simulink model "power_OLTCregtransformer"  (Simulink 6.0)
settings: Solver=ode23tb  StartTime=0.0  StopTime=120  MaxStep=1/60  RelTol=1e-4  AbsTol=1e-3
libraries: powerlib x75, powerlib_extras x18, simulink_extras x1
(part 2 of 3)

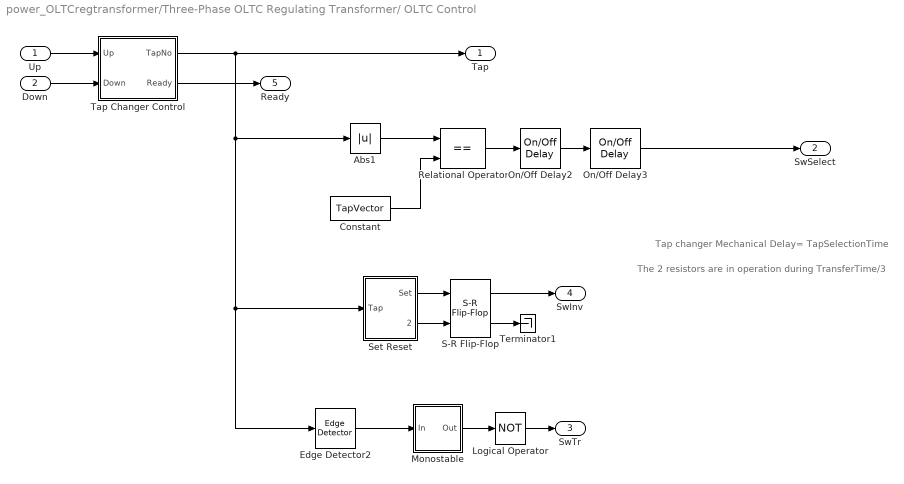
== system power_OLTCregtransformer/Three-Phase OLTC Regulating Transformer/ OLTC Control ==
  note: The 2 resistors are in operation during TransferTime/3
  note: Tap changer Mechanical Delay= TapSelectionTime
  Up : Inport  Port=1  LatchInput=off
  Down : Inport  Port=2  LatchInput=off
  Abs1 : Abs  SaturateOnIntegerOverflow=on
  Constant : Constant  Value=TapVector
  Edge Detector2 : powerlib_extras/Control  Blocks/Edge Detector  model=Either  ic=0
  Logical Operator : Logic  Operator=NOT  AllPortsSameDT=off
  Monostable : Subsystem  mask(Monostable Flip-Flop){EdgeDetect=Rising, t_mono=TransferTime, ic=1}
      mask prompts: EdgeDetect "Edge detection"; t_mono "Pulse duration (s):"; ic "Input at t = -eps:"
      mask help:
      | After being triggered  by the specified edge (Rising, Falling or Either), this block outputs a pulse (TRUE signal) for the time specified by parameter "Pulse duration".
      | If the specified edge is detected while the output is TRUE, the monostable is not retriggered
      |
      | The input value (0/1) at time preceeding t = 0 is specified by the parameter "input at t = -eps.
      mask init:
      | str=sprintf('%g %c',t_mono,'s');
      | if (EdgeDetect ~=3)
      |     x1 = (EdgeDetect -1)*10;
      |     x2 = (EdgeDetect -1)*30;
      | 	X1=[15-8,25,25,35+8]+0; Y1=[65+x2,65+x2,95-x2,95-x2];
      | 	X2=[15,25,35]+0;   Y2=[75+x1,85-x1,75+x1];
      | 	X3=[];X4=[];Y3=[];Y4=[];	
      | else
      | 	x1 = 10;
      | 	x2 = 30;
      | 	X1=[15,25,25,35]-14;  Y1=[65,65,95,95];
      | 	X2=[15,25,35]-14;    Y2=[75,85,75];
      | 	X3=[15,25,25,35]+14; Y3=[65+x2,65+x2,95-x2,95-x2];
      | 	X4=[15,25,35]+14;   Y4=[75+x1,85-x1,75+x1];
      | end
      mask StyleString: popup(Rising|Falling|Either),edit,edit
      mask Display:
      | plot(0,0,100,100,[100 75 75 25 25 0],[25 25 50 50 25 25]-0,X1,Y1,X2,Y2,X3,Y3,X4,Y4);
      | text(45,37,'T');
      | text(15,15,str);
  On/Off Delay2 : powerlib_extras/Control  Blocks/On//Off Delay  type_delay=On delay  delay=TransferTime/3  ic=1
  On/Off Delay3 : powerlib_extras/Control  Blocks/On//Off Delay  type_delay=Off delay  delay=2*TransferTime/3  ic=InitialStates
  Relational Operator : RelationalOperator  Operator===
  S-R Flip-Flop : simulink_extras/Flip Flops/S-R Flip-Flop  initial_condition=InitialTap>=0
  Set Reset : Subsystem
  Tap Changer Control : Subsystem  mask(Tap Changer Control){MinMaxTap=[-NumberOfTaps  +NumberOfTaps], InitialPosition=InitialTap, MecDelay=TapSelectionTime}
      mask prompts: MinMaxTap "Minimum and maximum tap number [ Min  Max ] :"; InitialPosition "Initial tap position"; MecDelay "Mechanical delay time"
      mask init:
      | if MecDelay<=0,
      | 	MecDelay=1/60;
      | end
  Terminator1 : Terminator
  Tap : Outport
  SwSelect : Outport  Port=2
  SwTr : Outport  Port=3
  SwInv : Outport  Port=4
  Ready : Outport  Port=5
  wires:
  On/Off Delay3/1 -> SwSelect/1
  Constant/1 -> Relational Operator/2
  Logical Operator/1 -> SwTr/1
  Down/1 -> Tap Changer Control/2(Down)
  Up/1 -> Tap Changer Control/1(Up)
  Relational Operator/1 -> On/Off Delay2/1
  On/Off Delay2/1 -> On/Off Delay3/1
  Monostable/1(Out) -> Logical Operator/1
  Tap Changer Control/1(TapNo) -> Tap/1, Edge Detector2/1, Set Reset/1(Tap), Abs1/1
  Tap Changer Control/2(Ready) -> Ready/1
  S-R Flip-Flop/2 -> Terminator1/1
  Set Reset/1(Set) -> S-R Flip-Flop/1
  Set Reset/2(Reset) -> S-R Flip-Flop/2
  Edge Detector2/1 -> Monostable/1(In)
  S-R Flip-Flop/1 -> SwInv/1
  Abs1/1 -> Relational Operator/1

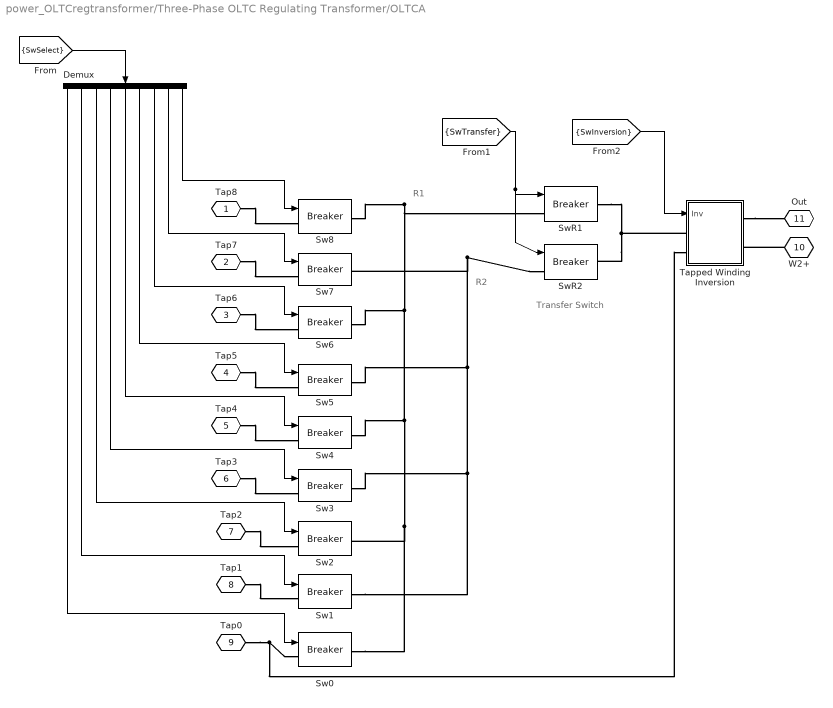
== system power_OLTCregtransformer/Three-Phase OLTC Regulating Transformer/OLTCA ==
  note: R2
  note: R1
  note: Transfer Switch
  Demux : Demux  Orientation=down  Outputs=9
  "Sw0 " : powerlib/Elements/Breaker  BreakerResistance=1e-4  InitialState=InitialStates(1)  SnubberResistance=1e6  SnubberCapacitance=inf  SwitchingTimes="[ 1/60  5/60 ]"  External=on  Measurements=None
  "Sw1 " : powerlib/Elements/Breaker  BreakerResistance=1e-4  InitialState=InitialStates(2)  SnubberResistance=1e6  SnubberCapacitance=inf  SwitchingTimes="[ 1/60  5/60 ]"  External=on  Measurements=None
  "Sw2 " : powerlib/Elements/Breaker  BreakerResistance=1e-4  InitialState=InitialStates(3)  SnubberResistance=1e6  SnubberCapacitance=inf  SwitchingTimes="[ 1/60  5/60 ]"  External=on  Measurements=None
  "Sw3 " : powerlib/Elements/Breaker  BreakerResistance=1e-4  InitialState=InitialStates(4)  SnubberResistance=1e6  SnubberCapacitance=inf  SwitchingTimes="[ 1/60  5/60 ]"  External=on  Measurements=None
  "Sw4 " : powerlib/Elements/Breaker  BreakerResistance=1e-4  InitialState=InitialStates(5)  SnubberResistance=1e6  SnubberCapacitance=inf  SwitchingTimes="[ 1/60  5/60 ]"  External=on  Measurements=None
  "Sw5 " : powerlib/Elements/Breaker  BreakerResistance=1e-4  InitialState=InitialStates(6)  SnubberResistance=1e6  SnubberCapacitance=inf  SwitchingTimes="[ 1/60  5/60 ]"  External=on  Measurements=None
  "Sw6 " : powerlib/Elements/Breaker  BreakerResistance=1e-4  InitialState=InitialStates(7)  SnubberResistance=1e6  SnubberCapacitance=inf  SwitchingTimes="[ 1/60  5/60 ]"  External=on  Measurements=None
  "Sw7 " : powerlib/Elements/Breaker  BreakerResistance=1e-4  InitialState=InitialStates(8)  SnubberResistance=1e6  SnubberCapacitance=inf  SwitchingTimes="[ 1/60  5/60 ]"  External=on  Measurements=None
  "Sw8 " : powerlib/Elements/Breaker  BreakerResistance=1e-4  InitialState=InitialStates(9)  SnubberResistance=1e6  SnubberCapacitance=inf  SwitchingTimes="[ 1/60  5/60 ]"  External=on  Measurements=None
  SwR1 : powerlib/Elements/Breaker  BreakerResistance=1e-4  InitialState=1  SnubberResistance=Rtransfer  SnubberCapacitance=inf  SwitchingTimes="[ 1/60  5/60 ]"  External=on  Measurements=None
  SwR2 : powerlib/Elements/Breaker  BreakerResistance=1e-4  InitialState=1  SnubberResistance=Rtransfer  SnubberCapacitance=inf  SwitchingTimes="[ 1/60  5/60 ]"  External=on  Measurements=None
  Tapped Winding Inversion : Subsystem
  Tap8 : PMIOPort  Port=1  Side=Right
  Tap7 : PMIOPort  Port=2  Side=Right
  Tap6 : PMIOPort  Port=3  Side=Right
  Tap5 : PMIOPort  Port=4  Side=Right
  Tap4 : PMIOPort  Port=5  Side=Right
  Tap3 : PMIOPort  Port=6  Side=Right
  Tap2 : PMIOPort  Port=7  Side=Right
  Tap1 : PMIOPort  Port=8  Side=Right
  Tap0 : PMIOPort  Port=9  Side=Right
  W2+ : PMIOPort  Orientation=left  Port=10  Side=Right
  Out : PMIOPort  Orientation=left  Port=11  Side=Left
  wires:
  Demux/9 -> "Sw8 "/1
  Demux/8 -> "Sw7 "/1
  Demux/7 -> "Sw6 "/1
  Demux/6 -> "Sw5 "/1
  Demux/5 -> "Sw4 "/1
  Demux/4 -> "Sw3 "/1
  Demux/3 -> "Sw2 "/1
  Demux/2 -> "Sw1 "/1
  Demux/1 -> "Sw0 "/1
  [SwInversion] -> Tapped Winding Inversion/1(Inv)
  [SwTransfer] -> SwR2/1, SwR1/1
  [SwSelect] -> Demux/1
  connections:
  "Sw0 "/LConn1 -- Tap0/RConn1 -- Tapped Winding Inversion/LConn2
  Tap1/RConn1 -- "Sw1 "/LConn1
  Tap2/RConn1 -- "Sw2 "/LConn1
  Tap6/RConn1 -- "Sw6 "/LConn1
  Tap4/RConn1 -- "Sw4 "/LConn1
  Tap5/RConn1 -- "Sw5 "/LConn1
  SwR1/RConn1 -- Tapped Winding Inversion/LConn1 -- SwR2/RConn1
  SwR2/LConn1 -- "Sw7 "/RConn1 -- "Sw5 "/RConn1 -- "Sw3 "/RConn1 -- "Sw1 "/RConn1
  Tapped Winding Inversion/RConn1 -- Out/RConn1
  W2+/RConn1 -- Tapped Winding Inversion/RConn2
  "Sw6 "/RConn1 -- "Sw4 "/RConn1 -- "Sw2 "/RConn1 -- "Sw0 "/RConn1 -- "Sw8 "/RConn1 -- SwR1/LConn1
  Tap3/RConn1 -- "Sw3 "/LConn1
  Tap8/RConn1 -- "Sw8 "/LConn1
  Tap7/RConn1 -- "Sw7 "/LConn1

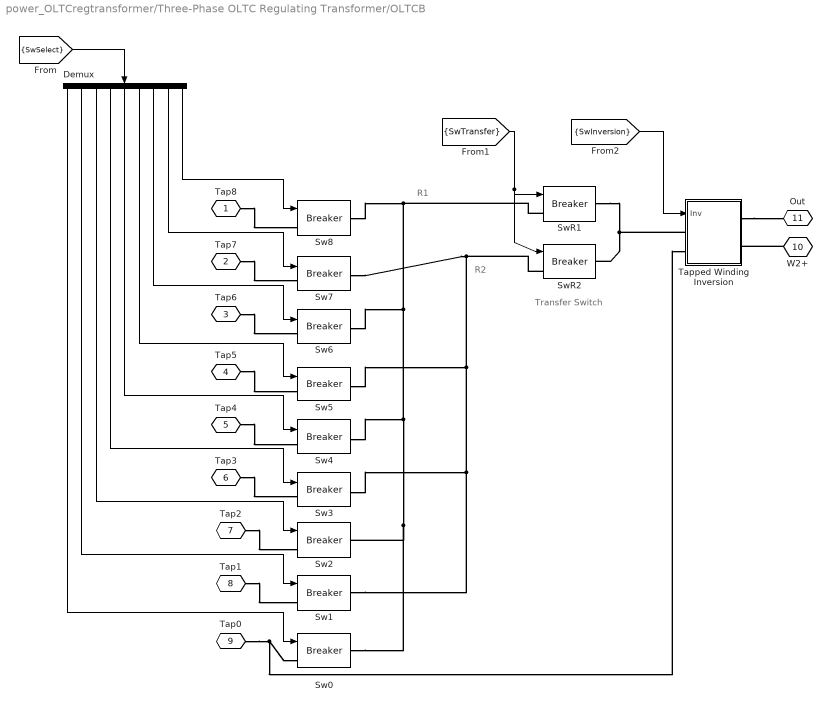
== system power_OLTCregtransformer/Three-Phase OLTC Regulating Transformer/OLTCB ==
  note: Transfer Switch
  note: R1
  note: R2
  Demux : Demux  Orientation=down  Outputs=9
  "Sw0 " : powerlib/Elements/Breaker  BreakerResistance=1e-4  InitialState=InitialStates(1)  SnubberResistance=1e6  SnubberCapacitance=inf  SwitchingTimes="[ 1/60  5/60 ]"  External=on  Measurements=None
  "Sw1 " : powerlib/Elements/Breaker  BreakerResistance=1e-4  InitialState=InitialStates(2)  SnubberResistance=1e6  SnubberCapacitance=inf  SwitchingTimes="[ 1/60  5/60 ]"  External=on  Measurements=None
  "Sw2 " : powerlib/Elements/Breaker  BreakerResistance=1e-4  InitialState=InitialStates(3)  SnubberResistance=1e6  SnubberCapacitance=inf  SwitchingTimes="[ 1/60  5/60 ]"  External=on  Measurements=None
  "Sw3 " : powerlib/Elements/Breaker  BreakerResistance=1e-4  InitialState=InitialStates(4)  SnubberResistance=1e6  SnubberCapacitance=inf  SwitchingTimes="[ 1/60  5/60 ]"  External=on  Measurements=None
  "Sw4 " : powerlib/Elements/Breaker  BreakerResistance=1e-4  InitialState=InitialStates(5)  SnubberResistance=1e6  SnubberCapacitance=inf  SwitchingTimes="[ 1/60  5/60 ]"  External=on  Measurements=None
  "Sw5 " : powerlib/Elements/Breaker  BreakerResistance=1e-4  InitialState=InitialStates(6)  SnubberResistance=1e6  SnubberCapacitance=inf  SwitchingTimes="[ 1/60  5/60 ]"  External=on  Measurements=None
  "Sw6 " : powerlib/Elements/Breaker  BreakerResistance=1e-4  InitialState=InitialStates(7)  SnubberResistance=1e6  SnubberCapacitance=inf  SwitchingTimes="[ 1/60  5/60 ]"  External=on  Measurements=None
  "Sw7 " : powerlib/Elements/Breaker  BreakerResistance=1e-4  InitialState=InitialStates(8)  SnubberResistance=1e6  SnubberCapacitance=inf  SwitchingTimes="[ 1/60  5/60 ]"  External=on  Measurements=None
  "Sw8 " : powerlib/Elements/Breaker  BreakerResistance=1e-4  InitialState=InitialStates(9)  SnubberResistance=1e6  SnubberCapacitance=inf  SwitchingTimes="[ 1/60  5/60 ]"  External=on  Measurements=None
  SwR1 : powerlib/Elements/Breaker  BreakerResistance=1e-4  InitialState=1  SnubberResistance=Rtransfer  SnubberCapacitance=inf  SwitchingTimes="[ 1/60  5/60 ]"  External=on  Measurements=None
  SwR2 : powerlib/Elements/Breaker  BreakerResistance=1e-4  InitialState=1  SnubberResistance=Rtransfer  SnubberCapacitance=inf  SwitchingTimes="[ 1/60  5/60 ]"  External=on  Measurements=None
  Tapped Winding Inversion : Subsystem
  Tap8 : PMIOPort  Port=1  Side=Right
  Tap7 : PMIOPort  Port=2  Side=Right
  Tap6 : PMIOPort  Port=3  Side=Right
  Tap5 : PMIOPort  Port=4  Side=Right
  Tap4 : PMIOPort  Port=5  Side=Right
  Tap3 : PMIOPort  Port=6  Side=Right
  Tap2 : PMIOPort  Port=7  Side=Right
  Tap1 : PMIOPort  Port=8  Side=Right
  Tap0 : PMIOPort  Port=9  Side=Right
  W2+ : PMIOPort  Orientation=left  Port=10  Side=Right
  Out : PMIOPort  Orientation=left  Port=11  Side=Left
  wires:
  [SwSelect] -> Demux/1
  [SwTransfer] -> SwR1/1, SwR2/1
  [SwInversion] -> Tapped Winding Inversion/1(Inv)
  Demux/1 -> "Sw0 "/1
  Demux/2 -> "Sw1 "/1
  Demux/3 -> "Sw2 "/1
  Demux/4 -> "Sw3 "/1
  Demux/5 -> "Sw4 "/1
  Demux/6 -> "Sw5 "/1
  Demux/7 -> "Sw6 "/1
  Demux/8 -> "Sw7 "/1
  Demux/9 -> "Sw8 "/1
  connections:
  Tap7/RConn1 -- "Sw7 "/LConn1
  Tap8/RConn1 -- "Sw8 "/LConn1
  Tap3/RConn1 -- "Sw3 "/LConn1
  "Sw0 "/RConn1 -- "Sw4 "/RConn1 -- SwR1/LConn1 -- "Sw8 "/RConn1 -- "Sw6 "/RConn1 -- "Sw2 "/RConn1
  W2+/RConn1 -- Tapped Winding Inversion/RConn2
  Tapped Winding Inversion/RConn1 -- Out/RConn1
  "Sw1 "/RConn1 -- "Sw3 "/RConn1 -- SwR2/LConn1 -- "Sw7 "/RConn1 -- "Sw5 "/RConn1
  SwR2/RConn1 -- Tapped Winding Inversion/LConn1 -- SwR1/RConn1
  Tap5/RConn1 -- "Sw5 "/LConn1
  Tap4/RConn1 -- "Sw4 "/LConn1
  Tap6/RConn1 -- "Sw6 "/LConn1
  Tap2/RConn1 -- "Sw2 "/LConn1
  Tap1/RConn1 -- "Sw1 "/LConn1
  "Sw0 "/LConn1 -- Tapped Winding Inversion/LConn2 -- Tap0/RConn1

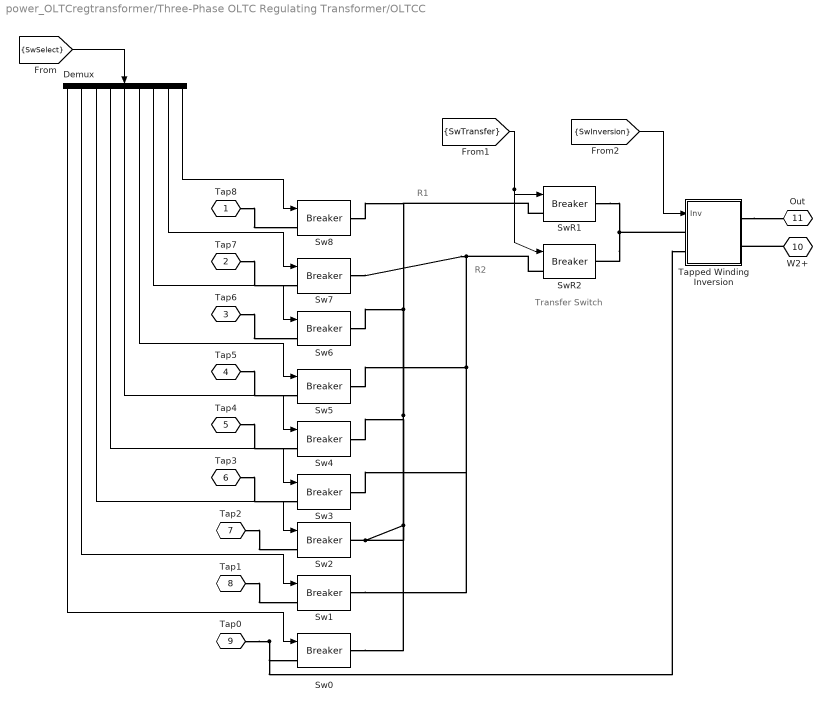
== system power_OLTCregtransformer/Three-Phase OLTC Regulating Transformer/OLTCC ==
  note: R2
  note: R1
  note: Transfer Switch
  Demux : Demux  Orientation=down  Outputs=9
  "Sw0 " : powerlib/Elements/Breaker  BreakerResistance=1e-4  InitialState=InitialStates(1)  SnubberResistance=1e6  SnubberCapacitance=inf  SwitchingTimes="[ 1/60  5/60 ]"  External=on  Measurements=None
  "Sw1 " : powerlib/Elements/Breaker  BreakerResistance=1e-4  InitialState=InitialStates(2)  SnubberResistance=1e6  SnubberCapacitance=inf  SwitchingTimes="[ 1/60  5/60 ]"  External=on  Measurements=None
  "Sw2 " : powerlib/Elements/Breaker  BreakerResistance=1e-4  InitialState=InitialStates(3)  SnubberResistance=1e6  SnubberCapacitance=inf  SwitchingTimes="[ 1/60  5/60 ]"  External=on  Measurements=None
  "Sw3 " : powerlib/Elements/Breaker  BreakerResistance=1e-4  InitialState=InitialStates(4)  SnubberResistance=1e6  SnubberCapacitance=inf  SwitchingTimes="[ 1/60  5/60 ]"  External=on  Measurements=None
  "Sw4 " : powerlib/Elements/Breaker  BreakerResistance=1e-4  InitialState=InitialStates(5)  SnubberResistance=1e6  SnubberCapacitance=inf  SwitchingTimes="[ 1/60  5/60 ]"  External=on  Measurements=None
  "Sw5 " : powerlib/Elements/Breaker  BreakerResistance=1e-4  InitialState=InitialStates(6)  SnubberResistance=1e6  SnubberCapacitance=inf  SwitchingTimes="[ 1/60  5/60 ]"  External=on  Measurements=None
  "Sw6 " : powerlib/Elements/Breaker  BreakerResistance=1e-4  InitialState=InitialStates(7)  SnubberResistance=1e6  SnubberCapacitance=inf  SwitchingTimes="[ 1/60  5/60 ]"  External=on  Measurements=None
  "Sw7 " : powerlib/Elements/Breaker  BreakerResistance=1e-4  InitialState=InitialStates(8)  SnubberResistance=1e6  SnubberCapacitance=inf  SwitchingTimes="[ 1/60  5/60 ]"  External=on  Measurements=None
  "Sw8 " : powerlib/Elements/Breaker  BreakerResistance=1e-4  InitialState=InitialStates(9)  SnubberResistance=1e6  SnubberCapacitance=inf  SwitchingTimes="[ 1/60  5/60 ]"  External=on  Measurements=None
  SwR1 : powerlib/Elements/Breaker  BreakerResistance=1e-4  InitialState=1  SnubberResistance=Rtransfer  SnubberCapacitance=inf  SwitchingTimes="[ 1/60  5/60 ]"  External=on  Measurements=None
  SwR2 : powerlib/Elements/Breaker  BreakerResistance=1e-4  InitialState=1  SnubberResistance=Rtransfer  SnubberCapacitance=inf  SwitchingTimes="[ 1/60  5/60 ]"  External=on  Measurements=None
  Tapped Winding Inversion : Subsystem
  Tap8 : PMIOPort  Port=1  Side=Right
  Tap7 : PMIOPort  Port=2  Side=Right
  Tap6 : PMIOPort  Port=3  Side=Right
  Tap5 : PMIOPort  Port=4  Side=Right
  Tap4 : PMIOPort  Port=5  Side=Right
  Tap3 : PMIOPort  Port=6  Side=Right
  Tap2 : PMIOPort  Port=7  Side=Right
  Tap1 : PMIOPort  Port=8  Side=Right
  Tap0 : PMIOPort  Port=9  Side=Right
  W2+ : PMIOPort  Orientation=left  Port=10  Side=Right
  Out : PMIOPort  Orientation=left  Port=11  Side=Left
  wires:
  Demux/9 -> "Sw8 "/1
  Demux/8 -> "Sw7 "/1
  Demux/7 -> "Sw6 "/1
  Demux/6 -> "Sw5 "/1
  Demux/5 -> "Sw4 "/1
  Demux/4 -> "Sw3 "/1
  Demux/3 -> "Sw2 "/1
  Demux/2 -> "Sw1 "/1
  Demux/1 -> "Sw0 "/1
  [SwInversion] -> Tapped Winding Inversion/1(Inv)
  [SwTransfer] -> SwR2/1, SwR1/1
  [SwSelect] -> Demux/1
  connections:
  Tap0/RConn1 -- Tapped Winding Inversion/LConn2 -- "Sw0 "/LConn1
  Tap1/RConn1 -- "Sw1 "/LConn1
  Tap2/RConn1 -- "Sw2 "/LConn1
  Tap6/RConn1 -- "Sw6 "/LConn1
  Tap4/RConn1 -- "Sw4 "/LConn1
  Tap5/RConn1 -- "Sw5 "/LConn1
  SwR1/RConn1 -- Tapped Winding Inversion/LConn1 -- SwR2/RConn1
  "Sw5 "/RConn1 -- "Sw7 "/RConn1 -- SwR2/LConn1 -- "Sw3 "/RConn1 -- "Sw1 "/RConn1
  Tapped Winding Inversion/RConn1 -- Out/RConn1
  W2+/RConn1 -- Tapped Winding Inversion/RConn2
  "Sw2 "/RConn1 -- "Sw6 "/RConn1 -- "Sw8 "/RConn1 -- SwR1/LConn1 -- "Sw4 "/RConn1 -- "Sw0 "/RConn1
  Tap3/RConn1 -- "Sw3 "/LConn1
  Tap8/RConn1 -- "Sw8 "/LConn1
  Tap7/RConn1 -- "Sw7 "/LConn1

== system power_OLTCregtransformer/Three-Phase OLTC Regulating Transformer/Subsystem ==
  note: A) Open the Three-Phase OLTC Transformer  mask (use Edit/Edit mask)
      |      In Initialization section, modify 1st line as below:
      |                   NumberOfTaps=10;
      |
      | B) Open the TransformerA block dialog box inside the Three-Phase OLTC Transformer (use Edit/Look under mask)
      |      and change the 'Number of Taps' parameter  from 7 to 9 (adding two intermediate taps on upper left winding (winding 1)).
      |
      | C) Open the  OLTCA block inside the Three-Phase OLTC Transformer (use Edit/Look under mask) and make the following changes:
      |       1) Open the dialog box of the Demux block and change the parameter  'Number of outputs' from 9 to 11.
      |       2) Add 2 switches labeled Sw9 and Sw10 (duplicate Sw8 block); Position these two blocks on top of Sw8 block.
      |       3) Open the dialog box of Sw9 and Sw10 blocks and change the  parameter "Initial state" as follows:
      |              Sw9 --> InitialState(10)
      |              Sw10-->InitialState(11)
      |      4) Add two connection ports labeled  respectively Tap9 and Tap10 (duplicate Tap8 block). Position these two blocks on top of Tap8 block.
      |      5) Renumber ALL connection ports as follows:
      |         Open dialog box of each connection port and change  'Port number' and  'Port location' parameters as in the the table below.
      |         (all port locations should be set to  'right' except for 'Out' port which must be 'left')
      |         Start the renumbering with the top port  labeled Tap10.
      |
      |            Port           Port          Port
      |            label       number   location
      |           ---------    -----------    -----------
      |            Tap10       1               right
      |            Tap9         2               right
      |            .....            ......              .......
      |            Tap 1       11               right
      |            Tap 0       12               right
      |            W2+         13               right
      |            Out           14               left
      |
      |     6) Connect terminal 1 of Sw9 and Sw10 respectively to ports labeled Tap10 (port #1)  and Tap9  (port #2)
      |     7) Connect terminal 2 of Sw9 and Sw10 respectively to nodes labeled R2 and R1
      |     8) Close the OLTCA block.
      |
      | D)  Connect the Tap10, Tap9 ...Tap0 connectors of OLTCA respectively to  1+, 1.1,   ... 1 connectors of tapped winding of TransformerA.
      |
      | E)  Cut  the OLTCB and OLTCC blocks and replace them with a duplicate of OLTCA block.  Rename these two blocks OLTCB and OLTCC.
      |
      | F)  Cut  the TransformerB and TransformerC blocks and replace them with a duplicate of TransformerA block. Rename these two blocks TransformerB and TransformerC.
      |
      | G) Make connections between OLTC to Transformer for  phases B and C as for phase A.
      |
      | H) Ckeck that the secondary windings of  the three transformers are connected in Delta (D1)
  note: The following procedure explains how to increase the number of taps from 8 (17 OLTC positions)  to 10  (21 OLTC positions)
      |    If you want to decrease the number of taps, follow the reverse procedure (Change 'add' to ' cut'  and skip step C3).

== system power_OLTCregtransformer/Three-Phase OLTC Regulating Transformer/TransformerA ==
  NWindingsTransformer : PMComponent  PhysicalDomain=powersysdomain  LeftPortType=p1  RightPortType=p1  LConnTagsString=1|2|3|4|5|6|7|8|9|10|11  RConnTagsString=1|2
      mask Type: InnerPowersysBlock
  1+ : PMIOPort  Port=1  Side=Left
  1.1 : PMIOPort  Port=2  Side=Left
  1.2 : PMIOPort  Port=3  Side=Left
  1.3 : PMIOPort  Port=4  Side=Left
  1.4 : PMIOPort  Port=5  Side=Left
  1.5 : PMIOPort  Port=6  Side=Left
  1.6 : PMIOPort  Port=7  Side=Left
  1.7 : PMIOPort  Port=8  Side=Left
  1 : PMIOPort  Port=9  Side=Left
  2+ : PMIOPort  Port=10  Side=Left
  2 : PMIOPort  Port=11  Side=Left
  +3 : PMIOPort  Orientation=left  Port=12  Side=Right
  3 : PMIOPort  Orientation=left  Port=13  Side=Right
  connections:
  NWindingsTransformer/RConn2 -- 3/RConn1
  NWindingsTransformer/RConn1 -- +3/RConn1
  1+/RConn1 -- NWindingsTransformer/LConn1
  NWindingsTransformer/LConn2 -- 1.1/RConn1
  NWindingsTransformer/LConn3 -- 1.2/RConn1
  NWindingsTransformer/LConn11 -- 2/RConn1
  NWindingsTransformer/LConn10 -- 2+/RConn1
  NWindingsTransformer/LConn9 -- 1/RConn1
  NWindingsTransformer/LConn4 -- 1.3/RConn1
  NWindingsTransformer/LConn5 -- 1.4/RConn1
  NWindingsTransformer/LConn6 -- 1.5/RConn1
  NWindingsTransformer/LConn7 -- 1.6/RConn1
  NWindingsTransformer/LConn8 -- 1.7/RConn1

== system power_OLTCregtransformer/Three-Phase OLTC Regulating Transformer/TransformerB ==
  NWindingsTransformer : PMComponent  PhysicalDomain=powersysdomain  LeftPortType=p1  RightPortType=p1  LConnTagsString=1|2|3|4|5|6|7|8|9|10|11  RConnTagsString=1|2
      mask Type: InnerPowersysBlock
  1+ : PMIOPort  Port=1  Side=Left
  1.1 : PMIOPort  Port=2  Side=Left
  1.2 : PMIOPort  Port=3  Side=Left
  1.3 : PMIOPort  Port=4  Side=Left
  1.4 : PMIOPort  Port=5  Side=Left
  1.5 : PMIOPort  Port=6  Side=Left
  1.6 : PMIOPort  Port=7  Side=Left
  1.7 : PMIOPort  Port=8  Side=Left
  1 : PMIOPort  Port=9  Side=Left
  2+ : PMIOPort  Port=10  Side=Left
  2 : PMIOPort  Port=11  Side=Left
  +3 : PMIOPort  Orientation=left  Port=12  Side=Right
  3 : PMIOPort  Orientation=left  Port=13  Side=Right
  connections:
  NWindingsTransformer/LConn8 -- 1.7/RConn1
  NWindingsTransformer/LConn7 -- 1.6/RConn1
  NWindingsTransformer/LConn6 -- 1.5/RConn1
  NWindingsTransformer/LConn5 -- 1.4/RConn1
  NWindingsTransformer/LConn4 -- 1.3/RConn1
  NWindingsTransformer/LConn9 -- 1/RConn1
  NWindingsTransformer/LConn10 -- 2+/RConn1
  NWindingsTransformer/LConn11 -- 2/RConn1
  NWindingsTransformer/LConn3 -- 1.2/RConn1
  NWindingsTransformer/LConn2 -- 1.1/RConn1
  1+/RConn1 -- NWindingsTransformer/LConn1
  NWindingsTransformer/RConn1 -- +3/RConn1
  NWindingsTransformer/RConn2 -- 3/RConn1

== system power_OLTCregtransformer/Three-Phase OLTC Regulating Transformer/TransformerC ==
  NWindingsTransformer : PMComponent  PhysicalDomain=powersysdomain  LeftPortType=p1  RightPortType=p1  LConnTagsString=1|2|3|4|5|6|7|8|9|10|11  RConnTagsString=1|2
      mask Type: InnerPowersysBlock
  1+ : PMIOPort  Port=1  Side=Left
  1.1 : PMIOPort  Port=2  Side=Left
  1.2 : PMIOPort  Port=3  Side=Left
  1.3 : PMIOPort  Port=4  Side=Left
  1.4 : PMIOPort  Port=5  Side=Left
  1.5 : PMIOPort  Port=6  Side=Left
  1.6 : PMIOPort  Port=7  Side=Left
  1.7 : PMIOPort  Port=8  Side=Left
  1 : PMIOPort  Port=9  Side=Left
  2+ : PMIOPort  Port=10  Side=Left
  2 : PMIOPort  Port=11  Side=Left
  +3 : PMIOPort  Orientation=left  Port=12  Side=Right
  3 : PMIOPort  Orientation=left  Port=13  Side=Right
  connections:
  NWindingsTransformer/RConn2 -- 3/RConn1
  NWindingsTransformer/RConn1 -- +3/RConn1
  1+/RConn1 -- NWindingsTransformer/LConn1
  NWindingsTransformer/LConn2 -- 1.1/RConn1
  NWindingsTransformer/LConn3 -- 1.2/RConn1
  NWindingsTransformer/LConn11 -- 2/RConn1
  NWindingsTransformer/LConn10 -- 2+/RConn1
  NWindingsTransformer/LConn9 -- 1/RConn1
  NWindingsTransformer/LConn4 -- 1.3/RConn1
  NWindingsTransformer/LConn5 -- 1.4/RConn1
  NWindingsTransformer/LConn6 -- 1.5/RConn1
  NWindingsTransformer/LConn7 -- 1.6/RConn1
  NWindingsTransformer/LConn8 -- 1.7/RConn1

== system power_OLTCregtransformer/Three-Phase OLTC Regulating Transformer/Voltage regulator ==
  Vmes (pu) : Inport  Port=1  LatchInput=off
  Ready : Inport  Port=2  LatchInput=off
  RegOn : Inport  Port=3  LatchInput=off
  Dead Zone : DeadZone  LowerValue=-DeadBand/2  UpperValue=+DeadBand/2  SaturateOnIntegerOverflow=on
  Logical Operator : Logic  AllPortsSameDT=off
  Logical Operator1 : Logic  AllPortsSameDT=off
  On/Off Delay : powerlib_extras/Control  Blocks/On//Off Delay  type_delay=On delay  delay=TimeDelay  ic=0
  On/Off Delay1 : powerlib_extras/Control  Blocks/On//Off Delay  type_delay=On delay  delay=TimeDelay  ic=0
  Relational Operator : RelationalOperator  Operator=<
  Relational Operator1 : RelationalOperator  Operator=>
  Sum : Sum  Inputs=|+-  SaturateOnIntegerOverflow=on
  Switch : Switch  Threshold=1.5  SaturateOnIntegerOverflow=on
  Transport Delay : TransportDelay  DelayTime=3/60  InitialInput=1
  Vref : Constant  Value=Vref
  Vref1 : Constant  Value=0
  Vref2 : Constant  Value=0
  Vref3 : Constant  Value=0
  Up : Outport
  Down : Outport  Port=2
  wires:
  Vref2/1 -> Switch/3
  RegOn/1 -> Switch/2
  Switch/1 -> Dead Zone/1
  Sum/1 -> Switch/1
  Vref/1 -> Sum/1
  Vmes (pu)/1 -> Sum/2
  Dead Zone/1 -> Relational Operator1/1, Relational Operator/1
  Vref1/1 -> Relational Operator/2
  Relational Operator/1 -> Logical Operator/1
  Ready/1 -> Transport Delay/1
  Logical Operator/1 -> On/Off Delay/1
  Transport Delay/1 -> Logical Operator/2, Logical Operator1/1
  On/Off Delay/1 -> Up/1
  Vref3/1 -> Relational Operator1/2
  Relational Operator1/1 -> Logical Operator1/2
  Logical Operator1/1 -> On/Off Delay1/1
  On/Off Delay1/1 -> Down/1

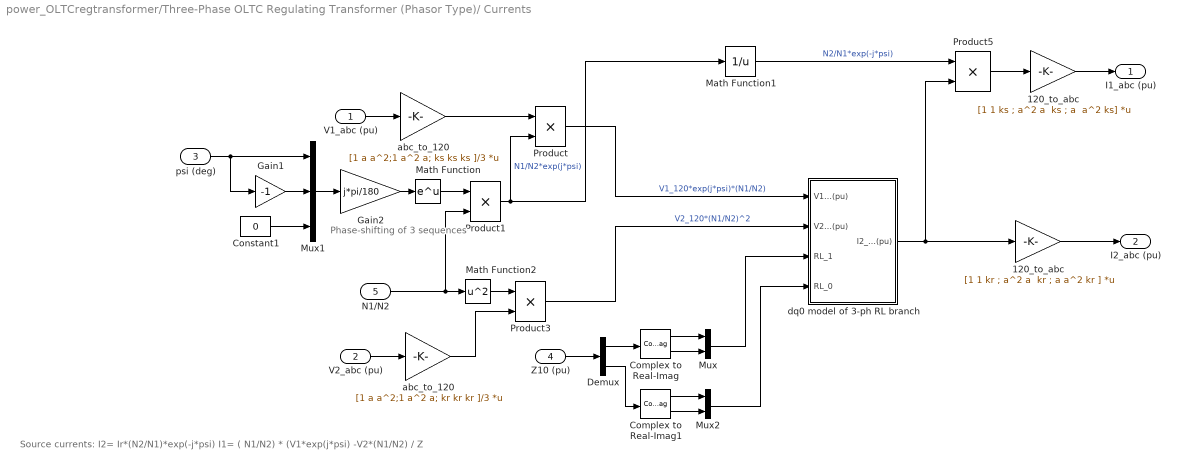
== system power_OLTCregtransformer/Three-Phase OLTC Regulating Transformer (Phasor Type)/ Currents  ==
  note: Source currents:
      |
      | I2= Ir*(N2/N1)*exp(-j*psi)
      | I1= ( N1/N2) * (V1*exp(j*psi) -V2*(N1/N2) / Z
  note: Phase-shifting
      | of 3 sequences
  V1_abc (pu) : Inport  Port=1  LatchInput=off
  V2_abc (pu) : Inport  Port=2  LatchInput=off
  psi (deg) : Inport  Port=3  LatchInput=off
  Z10 (pu) : Inport  Port=4  LatchInput=off
  N1/N2 : Inport  Port=5  LatchInput=off
  120_to_abc : Gain  Gain="[1 1 kr ; a^2 a  kr ; a a^2 kr ]"  Multiplication=Matrix(K*u)  SaturateOnIntegerOverflow=on
  "120_to_abc " : Gain  Gain="[1 1 ks ; a^2 a  ks ; a  a^2 ks]"  Multiplication=Matrix(K*u)  SaturateOnIntegerOverflow=on
  Complex to Real-Imag : ComplexToRealImag
  Complex to Real-Imag1 : ComplexToRealImag
  Constant1 : Constant  Value=0
  Demux : Demux  Outputs=2
  Gain1 : Gain  Gain=-1  SaturateOnIntegerOverflow=on
  Gain2 : Gain  Gain=j*pi/180  SaturateOnIntegerOverflow=on
  Math Function : Math  SaturateOnIntegerOverflow=on
  Math Function1 : Math  Operator=reciprocal  SaturateOnIntegerOverflow=on
  Math Function2 : Math  Operator=square  SaturateOnIntegerOverflow=on
  Mux : Mux  Inputs=2
  Mux1 : Mux  Inputs=3
  Mux2 : Mux  Inputs=2
  Product : Product  SaturateOnIntegerOverflow=on
  Product1 : Product  Inputs=**  SaturateOnIntegerOverflow=on
  Product3 : Product  Inputs=**  SaturateOnIntegerOverflow=on
  Product5 : Product  SaturateOnIntegerOverflow=on
  abc_to_120 : Gain  Gain=[1 a a^2;1 a^2 a; ks ks ks ]/3  Multiplication=Matrix(K*u)  SaturateOnIntegerOverflow=on
  "abc_to_120 " : Gain  Gain=[1 a a^2;1 a^2 a; kr kr kr ]/3  Multiplication=Matrix(K*u)  SaturateOnIntegerOverflow=on
  dq0 model of 3-ph RL branch : Subsystem
  I1_abc (pu) : Outport
  "I2_abc (pu) " : Outport  Port=2
  wires:
  Math Function2/1 -> Product3/1
  dq0 model of 3-ph RL branch/1(I2_120 (pu)) -> Product5/2, 120_to_abc/1
  Mux2/1 -> dq0 model of 3-ph RL branch/4(RL_0)
  Complex to Real-Imag1/2 -> Mux2/2
  Complex to Real-Imag1/1 -> Mux2/1
  Mux/1 -> dq0 model of 3-ph RL branch/3(RL_1)
  Complex to Real-Imag/2 -> Mux/2
  Complex to Real-Imag/1 -> Mux/1
  Demux/2 -> Complex to Real-Imag1/1
  Demux/1 -> Complex to Real-Imag/1
  Z10 (pu)/1 -> Demux/1
  "120_to_abc "/1 -> I1_abc (pu)/1
  120_to_abc/1 -> "I2_abc (pu) "/1
  "abc_to_120 "/1 -> Product3/2
  Constant1/1 -> Mux1/3
  Gain1/1 -> Mux1/2
  Mux1/1 -> Gain2/1
  psi (deg)/1 -> Mux1/1, Gain1/1
  Math Function1/1 -> Product5/1  "N2/N1*exp(-j*psi)"
  abc_to_120/1 -> Product/1
  Product5/1 -> "120_to_abc "/1
  V2_abc (pu)/1 -> "abc_to_120 "/1
  V1_abc (pu)/1 -> abc_to_120/1
  Math Function/1 -> Product1/1
  Product1/1 -> Product/2, Math Function1/1  "N1/N2*exp(j*psi)"
  N1/N2/1 -> Math Function2/1, Product1/2
  Product3/1 -> dq0 model of 3-ph RL branch/2(V2_120(pu))  "V2_120*(N1/N2)^2"
  Product/1 -> dq0 model of 3-ph RL branch/1(V1_120(pu))  "V1_120*exp(j*psi)*(N1/N2)"
  Gain2/1 -> Math Function/1

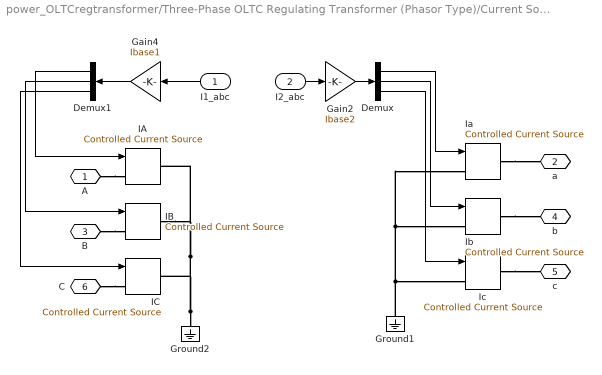
== system power_OLTCregtransformer/Three-Phase OLTC Regulating Transformer (Phasor Type)/Current Sources ==
  I1_abc : Inport  Orientation=left  Port=1  LatchInput=off
  I2_abc : Inport  Port=2  LatchInput=off
  Demux : Demux  Outputs=3
  Demux1 : Demux  Orientation=left  Outputs=3
  Gain2 : Gain  Gain=Ibase2  SaturateOnIntegerOverflow=on
  Gain4 : Gain  Orientation=left  Gain=Ibase1  SaturateOnIntegerOverflow=on
  Ground1 : powerlib/Elements/Ground  Orientation=down  PhysicalDomain=powersysdomain  SubClassName=unknown  LeftPortType=p1  RightPortType=p1  LConnTagsString=a
  Ground2 : powerlib/Elements/Ground  Orientation=down  PhysicalDomain=powersysdomain  SubClassName=unknown  LeftPortType=p1  RightPortType=p1  LConnTagsString=a
  IA : powerlib/Electrical Sources/Controlled Current Source  Initialize=on  Amplitude=Iw1A_init_mag  Phase=Iw1A_init_pha  Frequency=Fnom  Measurements=None
  IB : powerlib/Electrical Sources/Controlled Current Source  Initialize=on  Amplitude=Iw1B_init_mag  Phase=Iw1B_init_pha  Frequency=Fnom  Measurements=None
  IC : powerlib/Electrical Sources/Controlled Current Source  Initialize=on  Amplitude=Iw1C_init_mag  Phase=Iw1C_init_pha  Frequency=Fnom  Measurements=None
  Ia : powerlib/Electrical Sources/Controlled Current Source  Initialize=on  Amplitude=Iw2A_init_mag  Phase=Iw2A_init_pha  Frequency=Fnom  Measurements=None
  Ib : powerlib/Electrical Sources/Controlled Current Source  Initialize=on  Amplitude=Iw2B_init_mag  Phase=Iw2B_init_pha  Frequency=Fnom  Measurements=None
  Ic : powerlib/Electrical Sources/Controlled Current Source  Initialize=on  Amplitude=Iw2C_init_mag  Phase=Iw2C_init_pha  Frequency=Fnom  Measurements=None
  A : PMIOPort  Port=1  Side=Left
  a : PMIOPort  Orientation=left  Port=2  Side=Right
  B : PMIOPort  Port=3  Side=Left
  b : PMIOPort  Orientation=left  Port=4  Side=Right
  c : PMIOPort  Orientation=left  Port=5  Side=Right
  C : PMIOPort  Port=6  Side=Left
  wires:
  Gain4/1 -> Demux1/1
  Gain2/1 -> Demux/1
  Demux1/1 -> IA/1
  Demux1/2 -> IB/1
  Demux1/3 -> IC/1
  Demux/1 -> Ia/1
  Demux/2 -> Ib/1
  Demux/3 -> Ic/1
  I2_abc/1 -> Gain2/1
  I1_abc/1 -> Gain4/1
  connections:
  Ground2/LConn1 -- IC/RConn1 -- IA/RConn1 -- IB/RConn1
  Ground1/LConn1 -- Ic/LConn1 -- Ib/LConn1 -- Ia/LConn1
  A/RConn1 -- IA/LConn1
  B/RConn1 -- IB/LConn1
  C/RConn1 -- IC/LConn1
  Ia/RConn1 -- a/RConn1
  Ib/RConn1 -- b/RConn1
  Ic/RConn1 -- c/RConn1

== system power_OLTCregtransformer/Three-Phase OLTC Regulating Transformer (Phasor Type)/Tap Changer Control ==
  Up : Inport  Port=1  LatchInput=off
  Down : Inport  Port=2  LatchInput=off
  Constant : Constant  Value=-1
  Constant1 : Constant
  Determine tap positon : Subsystem
  Edge Detector : powerlib_extras/Control  Blocks/Edge Detector  model=Rising  ic=0
  Logical Operator : Logic  Operator=OR  AllPortsSameDT=off
  Logical Operator1 : Logic  AllPortsSameDT=off
  Mechanical Delay : TransportDelay  DelayTime=MecDelay  InitialInput=InitialPosition
  Memory : Memory  Orientation=left  X0=1  InheritSampleTime=on
  Relational Operator : RelationalOperator  Operator===  LogicOutDataTypeMode=Specify via dialog  LogicDataType=float('double')
  Switch : Switch  Threshold=0.5  SaturateOnIntegerOverflow=on
  TapNo : Outport
  Ready : Outport  Port=2
  wires:
  Mechanical Delay/1 -> TapNo/1, Relational Operator/2
  Logical Operator1/1 -> Determine tap positon/Trigger
  Up/1 -> Logical Operator/1
  Down/1 -> Logical Operator/2, Switch/2
  Constant/1 -> Switch/1
  Constant1/1 -> Switch/3
  Switch/1 -> Determine tap positon/1(NewTap)
  Determine tap positon/1(TapNo) -> Mechanical Delay/1, Relational Operator/1
  Relational Operator/1 -> Memory/1
  Memory/1 -> Logical Operator1/1, Ready/1
  Logical Operator/1 -> Edge Detector/1
  Edge Detector/1 -> Logical Operator1/2

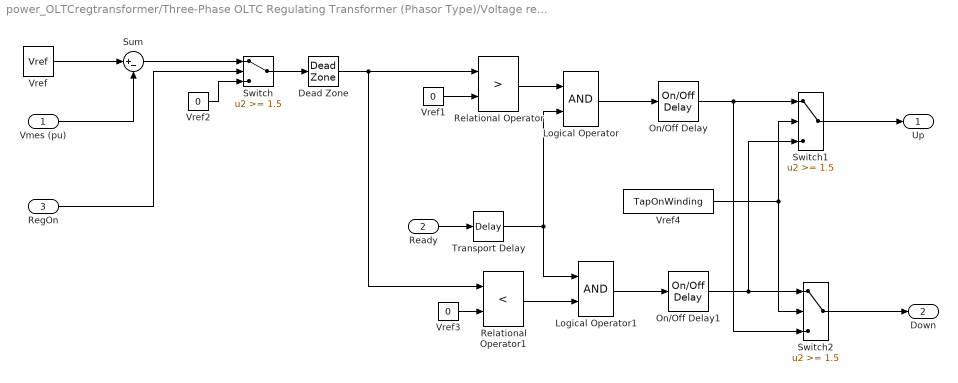
== system power_OLTCregtransformer/Three-Phase OLTC Regulating Transformer (Phasor Type)/Voltage regulator ==
  Vmes (pu) : Inport  Port=1  LatchInput=off
  Ready : Inport  Port=2  LatchInput=off
  RegOn : Inport  Port=3  LatchInput=off
  Dead Zone : DeadZone  LowerValue=-DeadBand/2  UpperValue=+DeadBand/2  SaturateOnIntegerOverflow=on
  Logical Operator : Logic  AllPortsSameDT=off
  Logical Operator1 : Logic  AllPortsSameDT=off
  On/Off Delay : powerlib_extras/Control  Blocks/On//Off Delay  type_delay=On delay  delay=TimeDelay  ic=0
  On/Off Delay1 : powerlib_extras/Control  Blocks/On//Off Delay  type_delay=On delay  delay=TimeDelay  ic=0
  Relational Operator : RelationalOperator  Operator=>
  Relational Operator1 : RelationalOperator  Operator=<
  Sum : Sum  Inputs=|+-  SaturateOnIntegerOverflow=on
  Switch : Switch  Threshold=1.5  SaturateOnIntegerOverflow=on
  Switch1 : Switch  Threshold=1.5  SaturateOnIntegerOverflow=on
  Switch2 : Switch  Threshold=1.5  SaturateOnIntegerOverflow=on
  Transport Delay : TransportDelay  DelayTime=3/60  InitialInput=1
  Vref : Constant  Value=Vref
  Vref1 : Constant  Value=0
  Vref2 : Constant  Value=0
  Vref3 : Constant  Value=0
  Vref4 : Constant  Value=TapOnWinding
  Up : Outport
  Down : Outport  Port=2
  wires:
  Logical Operator1/1 -> On/Off Delay1/1
  Relational Operator1/1 -> Logical Operator1/2
  Vref3/1 -> Relational Operator1/2
  Transport Delay/1 -> Logical Operator1/1, Logical Operator/2
  Logical Operator/1 -> On/Off Delay/1
  Ready/1 -> Transport Delay/1
  Relational Operator/1 -> Logical Operator/1
  Vref1/1 -> Relational Operator/2
  Dead Zone/1 -> Relational Operator/1, Relational Operator1/1
  Vmes (pu)/1 -> Sum/2
  Vref/1 -> Sum/1
  Sum/1 -> Switch/1
  Switch/1 -> Dead Zone/1
  RegOn/1 -> Switch/2
  Vref2/1 -> Switch/3
  On/Off Delay/1 -> Switch1/1, Switch2/3
  Switch1/1 -> Up/1
  On/Off Delay1/1 -> Switch2/1, Switch1/3
  Switch2/1 -> Down/1
  Vref4/1 -> Switch1/2, Switch2/2

== system power_OLTCregtransformer/Three-Phase OLTC Regulating Transformer (Phasor Type)/Z & Voltage Ratio ==
  note: Z10= vector of positive and zero-sequence impedances
      | psi= phase shift of  V2 with respect to V1 for positive-sequence
      | N2/N1 =  |V2|/|V1| = transformer ratio
      | N = nb of windings used at tap N
      | dU = voltage step  per tap (pu)
  Zw1 (pu) : Inport  Port=1  LatchInput=off
  Zw2 (pu) : Inport  Port=2  LatchInput=off
  Ztmax (pu) : Inport  Port=3  LatchInput=off
  TapNo : Inport  Port=4  LatchInput=off
  1st-Order  Filter4 : powerlib_extras/Control  Blocks/1st-Order  Filter  FilterType=Lowpass  Tc=1/Fnom  Initialize=on  Vac_Init="[0 0  Fnom]"  Vdc_Init=InitialTap  PlotResponse=off  param1=[1 500 1]
  Logical Operator : Logic  Operator=NOT  AllPortsSameDT=off
  Mux : Mux  Inputs=2
  RX1 : Constant  Value=TapOnWinding
  RX2 : Constant
  RX3 : Constant  Value=dU
  RX4 : Constant  Value=Nmax
  Relational Operator : RelationalOperator  Operator===
  Switch : Switch  Criteria=u2 ~= 0  Threshold=0.5  SaturateOnIntegerOverflow=on
  Switch1 : Switch  Criteria=u2 ~= 0  Threshold=0.5  SaturateOnIntegerOverflow=on
  Z Tap on winding 1 : Subsystem
  Z Tap on winding 2 : Subsystem
  "Z10 (pu) " : Outport
  N1/N2 : Outport  Port=2
  wires:
  Mux/1 -> "Z10 (pu) "/1
  Switch/1 -> Mux/2, Mux/1
  RX3/1 -> Z Tap on winding 2/2(dU), Z Tap on winding 1/2(dU)
  Ztmax (pu)/1 -> Z Tap on winding 2/5(Ztmax), Z Tap on winding 1/5(Ztmax)
  Switch1/1 -> N1/N2/1
  Z Tap on winding 2/2(N1/N2) -> Switch1/3
  Z Tap on winding 1/2(N1/N2) -> Switch1/1
  Z Tap on winding 2/1(Z) -> Switch/3
  Z Tap on winding 1/1(Z) -> Switch/1
  Logical Operator/1 -> Z Tap on winding 2/Enable
  Relational Operator/1 -> Switch1/2, Switch/2, Logical Operator/1, Z Tap on winding 1/Enable
  RX2/1 -> Relational Operator/2
  RX1/1 -> Relational Operator/1
  Zw1 (pu)/1 -> Z Tap on winding 2/3(Zw1), Z Tap on winding 1/3(Zw1)
  Zw2 (pu)/1 -> Z Tap on winding 2/4(Zw2), Z Tap on winding 1/4(Zw2)
  1st-Order  Filter4/1 -> Z Tap on winding 2/1(N), Z Tap on winding 1/1(N)  "N"
  TapNo/1 -> 1st-Order  Filter4/1  "N"
  RX4/1 -> Z Tap on winding 1/6(Nmax), Z Tap on winding 2/6(Nmax)

== system power_OLTCregtransformer/Three-Phase OLTC Regulating Transformer/ OLTC Control/Monostable ==
  note: Silvano Casoria
      | Power System Simulation Laboratory
      | IREQ, Hydro-Quebec
  note: Monostable
  In : Inport  Port=1  LatchInput=off
  Clock : Clock
      settings: Decimation=10
  Edge Detector : Subsystem  mask(Edge Detector){model=EdgeDetect, ic=ic}
      mask prompts: model "Edge:"; ic "Input at t = -eps:"
      mask help:
      | This block compares its present input to its previous input.
      |
      | If the input  is a logic signal (TRUE (1) or FALSE (0), the output is a one-step boolean signal TRUE  when  the specified edge (Rising, Falling or Either)  is detected.
      |
      | This block can also be used to detect the slope polarity of a continuous signal. For example, if the specified edge is  "Rising", the output is TRUE as long as the slope of the input signal is positive.
      |
      | The input value at time preceeding t=0 is specified by the parameter "Input at t=-eps"
      mask init:
      | if model~=3,
      | 	x1 = (model -1)*20;
      |     x2 = (model -1)*60;
      | 	X1=[5,20,20,35]+25; Y1=[20+x2,20+x2,80-x2,80-x2];
      | 	X2=[5,20,35]+25;    Y2=[40+x1,60-x1,40+x1];
      | 	X3=[];X4=[];Y3=[];Y4=[];
      | else
      | 	x1 = 20;
      | 	x2 = 60;
      | 	X1=[5,20,20,35]+8; Y1=[20,20,80,80];
      | 	X2=[5,20,35]+8;    Y2=[40,60,40];
      | 	X3=[5,20,20,35]+53; Y3=[20+x2,20+x2,80-x2,80-x2];
      | 	X4=[5,20,35]+53;    Y4=[40+x1,60-x1,40+x1];
      | end
      mask Display: plot(0,0,100,100, X1,Y1,X2,Y2,X3,Y3,X4,Y4);
  Logical Operator1 : Logic
  Logical Operator2 : Logic  Orientation=left  Operator=NOT  Inputs=1
  Memory : Memory  Orientation=left  InheritSampleTime=on
  Relational Operator : RelationalOperator  Operator=>  InputSameDT=on
  Sample & Hold : powerlib_extras/Control  Blocks/Sample & Hold  ic=-1e6
  Sum : Sum  SaturateOnIntegerOverflow=on  InputSameDT=on
  T_monostable : Constant  Value=t_mono - eps
  Out : Outport
  wires:
  Logical Operator1/1 -> Sample & Hold/2
  T_monostable/1 -> Sum/2
  Clock/1 -> Sample & Hold/1, Relational Operator/2
  Sum/1 -> Relational Operator/1
  Sample & Hold/1 -> Sum/1
  Memory/1 -> Logical Operator2/1
  Edge Detector/1(Out) -> Logical Operator1/2
  Logical Operator2/1 -> Logical Operator1/1
  Relational Operator/1 -> Memory/1, Out/1
  In/1 -> Edge Detector/1(In)

== system power_OLTCregtransformer/Three-Phase OLTC Regulating Transformer/ OLTC Control/Set Reset ==
  Tap : Inport  Port=1  LatchInput=off
  Constant1 : Constant  Value=-1
  Constant2 : Constant
  Edge Detector1 : powerlib_extras/Control  Blocks/Edge Detector  model=Rising  ic=0
  Edge Detector2 : powerlib_extras/Control  Blocks/Edge Detector  model=Falling  ic=0
  Logical Operator1 : Logic  AllPortsSameDT=off
  Logical Operator2 : Logic  AllPortsSameDT=off
  Relational Operator1 : RelationalOperator  Operator===
  Relational Operator2 : RelationalOperator  Operator===
  Set : Outport
  Reset : Outport  Port=2
  wires:
  Constant1/1 -> Relational Operator1/2
  Relational Operator1/1 -> Logical Operator2/2
  Edge Detector2/1 -> Logical Operator2/1
  Logical Operator2/1 -> Reset/1
  Tap/1 -> Edge Detector2/1, Relational Operator1/1, Edge Detector1/1, Relational Operator2/1
  Constant2/1 -> Relational Operator2/2
  Relational Operator2/1 -> Logical Operator1/2
  Edge Detector1/1 -> Logical Operator1/1
  Logical Operator1/1 -> Set/1

== system power_OLTCregtransformer/Three-Phase OLTC Regulating Transformer/ OLTC Control/Tap Changer Control ==
  Up : Inport  Port=1  LatchInput=off
  Down : Inport  Port=2  LatchInput=off
  Constant : Constant  Value=-1
  Constant1 : Constant
  Determine tap positon : Subsystem
  Edge Detector : powerlib_extras/Control  Blocks/Edge Detector  model=Rising  ic=0
  Logical Operator : Logic  Operator=OR  AllPortsSameDT=off
  Logical Operator1 : Logic  AllPortsSameDT=off
  Mechanical Delay : TransportDelay  DelayTime=MecDelay  InitialInput=InitialPosition
  Memory : Memory  Orientation=left  X0=1  InheritSampleTime=on
  Relational Operator : RelationalOperator  Operator===  LogicOutDataTypeMode=Specify via dialog  LogicDataType=float('double')
  Switch : Switch  Threshold=0.5  SaturateOnIntegerOverflow=on
  TapNo : Outport
  Ready : Outport  Port=2
  wires:
  Mechanical Delay/1 -> TapNo/1, Relational Operator/2
  Logical Operator1/1 -> Determine tap positon/Trigger
  Up/1 -> Logical Operator/1
  Down/1 -> Logical Operator/2, Switch/2
  Constant/1 -> Switch/1
  Constant1/1 -> Switch/3
  Switch/1 -> Determine tap positon/1(NewTap)
  Determine tap positon/1(TapNo) -> Mechanical Delay/1, Relational Operator/1
  Relational Operator/1 -> Memory/1
  Memory/1 -> Logical Operator1/1, Ready/1
  Logical Operator/1 -> Edge Detector/1
  Edge Detector/1 -> Logical Operator1/2

== system power_OLTCregtransformer/Three-Phase OLTC Regulating Transformer/OLTCA/Tapped Winding Inversion ==
  Inv : Inport  Port=1  LatchInput=off
  Logical Operator : Logic  Operator=NOT  AllPortsSameDT=off
  SwInv1 : powerlib/Elements/Breaker  BreakerResistance=1e-4  InitialState=InitialStateInv1  SnubberResistance=1e6  SnubberCapacitance=inf  SwitchingTimes="[ 1/60  5/60 ]"  External=on  Measurements=None
  SwInv2 : powerlib/Elements/Breaker  BreakerResistance=1e-4  InitialState=InitialStateInv2  SnubberResistance=1e6  SnubberCapacitance=inf  SwitchingTimes="[ 1/60  5/60 ]"  External=on  Measurements=None
  SwInv3 : powerlib/Elements/Breaker  BreakerResistance=1e-4  InitialState=InitialStateInv3  SnubberResistance=1e6  SnubberCapacitance=inf  SwitchingTimes="[ 1/60  5/60 ]"  External=on  Measurements=None
  SwInv4 : powerlib/Elements/Breaker  BreakerResistance=1e-4  InitialState=InitialStateInv4  SnubberResistance=1e6  SnubberCapacitance=inf  SwitchingTimes="[ 1/60  5/60 ]"  External=on  Measurements=None
  In1 : PMIOPort  Port=1  Side=Left
  In2 : PMIOPort  Port=2  Side=Left
  Out1 : PMIOPort  Orientation=left  Port=3  Side=Right
  Out2 : PMIOPort  Orientation=left  Port=4  Side=Right
  wires:
  Logical Operator/1 -> SwInv4/1, SwInv2/1
  Inv/1 -> Logical Operator/1, SwInv3/1, SwInv1/1
  connections:
  SwInv4/LConn1 -- SwInv3/LConn1 -- In2/RConn1
  Out2/RConn1 -- SwInv2/RConn1 -- SwInv3/RConn1
  SwInv2/LConn1 -- SwInv1/LConn1 -- In1/RConn1
  Out1/RConn1 -- SwInv4/RConn1 -- SwInv1/RConn1

== system power_OLTCregtransformer/Three-Phase OLTC Regulating Transformer/OLTCB/Tapped Winding Inversion ==
  Inv : Inport  Port=1  LatchInput=off
  Logical Operator : Logic  Operator=NOT  AllPortsSameDT=off
  SwInv1 : powerlib/Elements/Breaker  BreakerResistance=1e-4  InitialState=InitialStateInv1  SnubberResistance=1e6  SnubberCapacitance=inf  SwitchingTimes="[ 1/60  5/60 ]"  External=on  Measurements=None
  SwInv2 : powerlib/Elements/Breaker  BreakerResistance=1e-4  InitialState=InitialStateInv2  SnubberResistance=1e6  SnubberCapacitance=inf  SwitchingTimes="[ 1/60  5/60 ]"  External=on  Measurements=None
  SwInv3 : powerlib/Elements/Breaker  BreakerResistance=1e-4  InitialState=InitialStateInv3  SnubberResistance=1e6  SnubberCapacitance=inf  SwitchingTimes="[ 1/60  5/60 ]"  External=on  Measurements=None
  SwInv4 : powerlib/Elements/Breaker  BreakerResistance=1e-4  InitialState=InitialStateInv4  SnubberResistance=1e6  SnubberCapacitance=inf  SwitchingTimes="[ 1/60  5/60 ]"  External=on  Measurements=None
  In1 : PMIOPort  Port=1  Side=Left
  In2 : PMIOPort  Port=2  Side=Left
  Out1 : PMIOPort  Orientation=left  Port=3  Side=Right
  Out2 : PMIOPort  Orientation=left  Port=4  Side=Right
  wires:
  Inv/1 -> SwInv1/1, SwInv3/1, Logical Operator/1
  Logical Operator/1 -> SwInv2/1, SwInv4/1
  connections:
  SwInv1/RConn1 -- SwInv4/RConn1 -- Out1/RConn1
  In1/RConn1 -- SwInv1/LConn1 -- SwInv2/LConn1
  SwInv3/RConn1 -- SwInv2/RConn1 -- Out2/RConn1
  In2/RConn1 -- SwInv3/LConn1 -- SwInv4/LConn1

== system power_OLTCregtransformer/Three-Phase OLTC Regulating Transformer/OLTCC/Tapped Winding Inversion ==
  Inv : Inport  Port=1  LatchInput=off
  Logical Operator : Logic  Operator=NOT  AllPortsSameDT=off
  SwInv1 : powerlib/Elements/Breaker  BreakerResistance=1e-4  InitialState=InitialStateInv1  SnubberResistance=1e6  SnubberCapacitance=inf  SwitchingTimes="[ 1/60  5/60 ]"  External=on  Measurements=None
  SwInv2 : powerlib/Elements/Breaker  BreakerResistance=1e-4  InitialState=InitialStateInv2  SnubberResistance=1e6  SnubberCapacitance=inf  SwitchingTimes="[ 1/60  5/60 ]"  External=on  Measurements=None
  SwInv3 : powerlib/Elements/Breaker  BreakerResistance=1e-4  InitialState=InitialStateInv3  SnubberResistance=1e6  SnubberCapacitance=inf  SwitchingTimes="[ 1/60  5/60 ]"  External=on  Measurements=None
  SwInv4 : powerlib/Elements/Breaker  BreakerResistance=1e-4  InitialState=InitialStateInv4  SnubberResistance=1e6  SnubberCapacitance=inf  SwitchingTimes="[ 1/60  5/60 ]"  External=on  Measurements=None
  In1 : PMIOPort  Port=1  Side=Left
  In2 : PMIOPort  Port=2  Side=Left
  Out1 : PMIOPort  Orientation=left  Port=3  Side=Right
  Out2 : PMIOPort  Orientation=left  Port=4  Side=Right
  wires:
  Logical Operator/1 -> SwInv4/1, SwInv2/1
  Inv/1 -> Logical Operator/1, SwInv3/1, SwInv1/1
  connections:
  SwInv4/LConn1 -- SwInv3/LConn1 -- In2/RConn1
  Out2/RConn1 -- SwInv2/RConn1 -- SwInv3/RConn1
  SwInv2/LConn1 -- SwInv1/LConn1 -- In1/RConn1
  Out1/RConn1 -- SwInv4/RConn1 -- SwInv1/RConn1

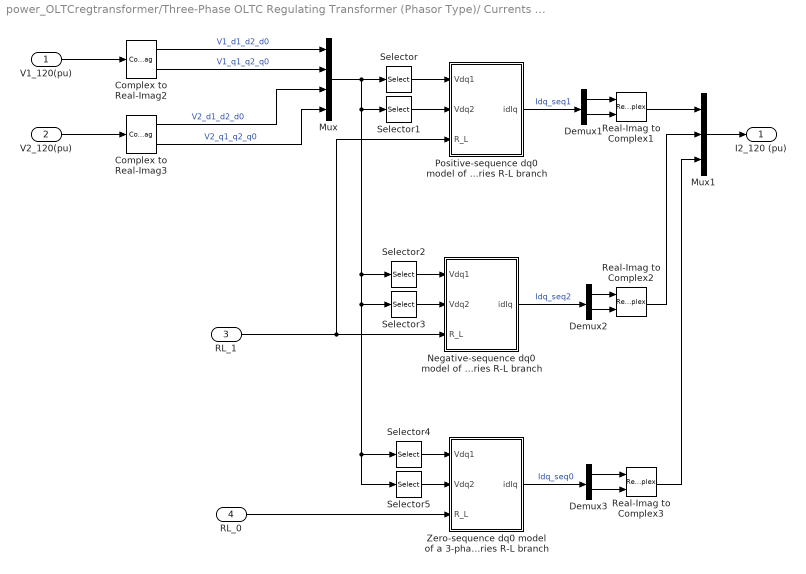
== system power_OLTCregtransformer/Three-Phase OLTC Regulating Transformer (Phasor Type)/ Currents /dq0 model of 3-ph RL branch ==
  V1_120(pu) : Inport  Port=1  LatchInput=off
  V2_120(pu) : Inport  Port=2  LatchInput=off
  RL_1 : Inport  Port=3  LatchInput=off
  RL_0 : Inport  Port=4  LatchInput=off
  Complex to Real-Imag2 : ComplexToRealImag
  Complex to Real-Imag3 : ComplexToRealImag
  Demux1 : Demux  Outputs=2
  Demux2 : Demux  Outputs=2
  Demux3 : Demux  Outputs=2
  Mux : Mux
  Mux1 : Mux  Inputs=3
  Negative-sequence dq0 model of a 3-phase series R-L branch : Subsystem
  Positive-sequence dq0 model of a 3-phase series R-L branch : Subsystem
  Real-Imag to Complex1 : RealImagToComplex
  Real-Imag to Complex2 : RealImagToComplex
  Real-Imag to Complex3 : RealImagToComplex
  Selector : Selector  Elements=[1 4]  InputPortWidth=12
  Selector1 : Selector  Elements=[7 10]  InputPortWidth=12
  Selector2 : Selector  Elements=[1 4]+1  InputPortWidth=12
  Selector3 : Selector  Elements=[7 10]+1  InputPortWidth=12
  Selector4 : Selector  Elements=[1 4]+2  InputPortWidth=12
  Selector5 : Selector  Elements=[7 10]+2  InputPortWidth=12
  Zero-sequence dq0 model of a 3-phase series R-L branch : Subsystem
  I2_120 (pu) : Outport
  wires:
  Mux1/1 -> I2_120 (pu)/1
  Real-Imag to Complex3/1 -> Mux1/3
  Demux3/1 -> Real-Imag to Complex3/1
  Demux3/2 -> Real-Imag to Complex3/2
  Real-Imag to Complex2/1 -> Mux1/2
  Demux2/1 -> Real-Imag to Complex2/1
  Demux2/2 -> Real-Imag to Complex2/2
  Real-Imag to Complex1/1 -> Mux1/1
  Demux1/1 -> Real-Imag to Complex1/1
  Demux1/2 -> Real-Imag to Complex1/2
  RL_0/1 -> Zero-sequence dq0 model of a 3-phase series R-L branch/3(R_L)
  Selector5/1 -> Zero-sequence dq0 model of a 3-phase series R-L branch/2(Vdq2)
  RL_1/1 -> Negative-sequence dq0 model of a 3-phase series R-L branch/3(R_L), Positive-sequence dq0 model of a 3-phase series R-L branch/3(R_L)
  Complex to Real-Imag3/2 -> Mux/4  "V2_q1_q2_q0"
  Complex to Real-Imag3/1 -> Mux/3  "V2_d1_d2_d0"
  Complex to Real-Imag2/2 -> Mux/2  "V1_q1_q2_q0"
  Complex to Real-Imag2/1 -> Mux/1  "V1_d1_d2_d0"
  Zero-sequence dq0 model of a 3-phase series R-L branch/1(idIq) -> Demux3/1  "Idq_seq0"
  Negative-sequence dq0 model of a 3-phase series R-L branch/1(idIq) -> Demux2/1  "Idq_seq2"
  Selector4/1 -> Zero-sequence dq0 model of a 3-phase series R-L branch/1(Vdq1)
  Selector3/1 -> Negative-sequence dq0 model of a 3-phase series R-L branch/2(Vdq2)
  Selector2/1 -> Negative-sequence dq0 model of a 3-phase series R-L branch/1(Vdq1)
  Mux/1 -> Selector5/1, Selector4/1, Selector3/1, Selector2/1, Selector1/1, Selector/1
  Selector1/1 -> Positive-sequence dq0 model of a 3-phase series R-L branch/2(Vdq2)
  Selector/1 -> Positive-sequence dq0 model of a 3-phase series R-L branch/1(Vdq1)
  V2_120(pu)/1 -> Complex to Real-Imag3/1
  V1_120(pu)/1 -> Complex to Real-Imag2/1
  Positive-sequence dq0 model of a 3-phase series R-L branch/1(idIq) -> Demux1/1  "Idq_seq1"

== system power_OLTCregtransformer/Three-Phase OLTC Regulating Transformer (Phasor Type)/Tap Changer Control/Determine tap positon ==
  NewTap : Inport  Port=1  LatchInput=off
  Trigger : TriggerPort
  Memory : Memory  Orientation=left  X0=InitialPosition  InheritSampleTime=on
  Saturation : Saturate  UpperLimit=MinMaxTap(2)  LowerLimit=MinMaxTap(1)
  Sum : Sum  Inputs=|++  SaturateOnIntegerOverflow=on
  TapNo : Outport  InitialOutput=InitialPosition
  wires:
  NewTap/1 -> Sum/1
  Sum/1 -> Saturation/1
  Memory/1 -> Sum/2
  Saturation/1 -> TapNo/1, Memory/1

== system power_OLTCregtransformer/Three-Phase OLTC Regulating Transformer (Phasor Type)/Z & Voltage Ratio/Z Tap on winding 1 ==
  note: Tap changer on winding 1:
      | Z = Z1  + Z2*(1+NdU)^2 +  Ztmax*N*Nmax*(dU)^2       (pu based on Pnom and V1nom)
      | N1/N2= 1+N*dU
      |
      | where :
      | Zw1   =  impedance of winding 1 (pu based on Pnom and V1nom)
      | Zw2   =  impedance of winding 2 (pu based on Pnom and V2nom)
      | Ztmax =   impedance of tapped winding at maximum tap (Nmax)     (pu  based on  Pnom & Nmax*dU)
      | Zt =  impedance of tapped winding at tap N
      |      = Ztmax*N/Nmax*(Nmax.dU)^2 = Ztmax*N*Nmax*(dU)^2              (pu based on Pnom and V1nom)
  N : Inport  Port=1  LatchInput=off
  dU : Inport  Port=2  LatchInput=off
  Zw1 : Inport  Port=3  LatchInput=off
  Zw2 : Inport  Port=4  LatchInput=off
  Ztmax : Inport  Port=5  LatchInput=off
  Nmax : Inport  Port=6  LatchInput=off
  Enable : EnablePort
  Math Function1 : Math  Operator=square  SaturateOnIntegerOverflow=on
  Math Function2 : Math  Operator=square  SaturateOnIntegerOverflow=on
  Product1 : Product  SaturateOnIntegerOverflow=on
  Product2 : Product  SaturateOnIntegerOverflow=on
  Product3 : Product  Inputs=****  SaturateOnIntegerOverflow=on
  Psi1 : Constant
  Sum1 : Sum  Inputs=+++  SaturateOnIntegerOverflow=on
  Sum2 : Sum  SaturateOnIntegerOverflow=on
  Z : Outport
  N1/N2 : Outport  Port=2
  wires:
  Product3/1 -> Sum1/1  "Zt = Ztmax*N*Nmax*(dU)^2"
  Product1/1 -> Sum2/1  "NdU"
  dU/1 -> Product1/2, Math Function1/1
  N/1 -> Product1/1, Product3/3
  Sum2/1 -> N1/N2/1, Math Function2/1  "1+NdU"
  Psi1/1 -> Sum2/2
  Zw1/1 -> Sum1/3
  Zw2/1 -> Product2/2
  Sum1/1 -> Z/1
  Math Function2/1 -> Product2/1
  Product2/1 -> Sum1/2
  Ztmax/1 -> Product3/1
  Math Function1/1 -> Product3/4
  Nmax/1 -> Product3/2
